simulink model "me132Hw1Q4_BallTrajectory"  (R2021a)
settings: Solver=VariableStepAuto  StartTime=0.0  StopTime=time_end  RelTol=1e-3
values from neighbouring files (symbols this model uses):
  g = -9.81    [hw1Q4.m]    (also in hw1Q5.m)
  mass = 0.3    [hw1Q4.m]    (also in hw1Q5.m)
  v0_x = 35 * cosd(65)    [hw1Q4.m]    (also in hw1Q5.m)
  v0_y = 35 * sind(65)    [hw1Q4.m]    (also in hw1Q5.m)
settings Model: Creator=kaiyu  LastModifiedBy=kaiyu

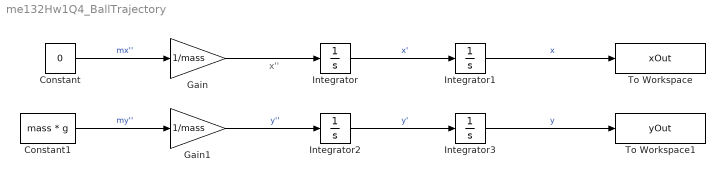
== system me132Hw1Q4_BallTrajectory ==
  note: x''
  Constant : Constant  Value=0
  Constant1 : Constant  Value=mass * g
  Gain : Gain  Gain=1/mass
  Gain1 : Gain  Gain=1/mass
  Integrator : Integrator  InitialCondition=v0_x
  Integrator1 : Integrator
  Integrator2 : Integrator  InitialCondition=v0_y
  Integrator3 : Integrator
  To Workspace : ToWorkspace  VariableName=xOut  SaveFormat=Timeseries  SampleTime=-1
  To Workspace1 : ToWorkspace  VariableName=yOut  SaveFormat=Timeseries  SampleTime=-1
  wires:
  Constant/1 -> Gain/1  "mx''"
  Constant1/1 -> Gain1/1  "my''"
  Integrator/1 -> Integrator1/1  "x'"
  Gain/1 -> Integrator/1
  Gain1/1 -> Integrator2/1  "y''"
  Integrator2/1 -> Integrator3/1  "y'"
  Integrator3/1 -> To Workspace1/1  "y"
  Integrator1/1 -> To Workspace/1  "x"
